simulink model "PMSM_FOC"  (R2015b)
settings: Solver=FixedStepDiscrete  StartTime=0.0  StopTime=0.3  RelTol=1e-3
PostLoadFcn:
  | PMSM_Params
undefined symbols (not defined in the file): Params, Plot_PMSM
libraries: powerlib x7
settings Model: Creator=Pascal  LastModifiedBy=reynaudp
settings DataIOCC: SaveFormat=Array
settings OptimizationCC: OptimizeModelRefInitCode=on  LifeSpan=1
settings DebuggingCC: UnderspecifiedInitializationDetection=Classic  MergeDetectMultiDrivingBlocksExec=none  SolverPrmCheckMsg=warning  StateNameClashWarn=warning
settings HardwareCC: ProdBitPerPointer=32  ProdLargestAtomicInteger=Integer  ProdWordSize=32  ProdHWDeviceType=STMicroelectronics->STM32 32-bit Cortex-M
settings RTWCC: SystemTargetFile=stm32.tlc  TemplateMakefile=stm32.tmf  Description=stm32 (Embedded Target)  GenerateReport=on  IncludeHyperlinkInReport=on  CodeExecutionProfiling=on  CodeProfilingSaveOptions=AllData  GenerateCodeReplacementReport=on
settings CodeAppCC: IgnoreCustomStorageClasses=off  MaxIdLength=64  CustomSymbolStrType=$N$R$M  SimulinkBlockComments=off  InternalIdentifier=Classic
settings STFCustomTargetCC: CodeReplacementLibrary=ARM CMSIS SIN COS  ParMdlRefBuildCompliant=on  ConcurrentExecutionCompliant=off  IncludeMdlTerminateFcn=off  GeneratePreprocessorConditionals=Use local settings  CombineOutputUpdateFcns=on  ERTCustomFileBanners=on  SupportContinuousTime=off  SupportNonInlinedSFcns=off  MATLABClassNameForMDSCustomization=Simulink.SoftwareTarget.ERTCustomization  CPPClassGenCompliant=off  GRTInterface=off  SystemTargetFile=stm32.tlc
settings ERTTargetCC: CodeReplacementLibrary=ARM CMSIS SIN COS  CompOptLevelCompliant=off  ConcurrentExecutionCompliant=off  IncludeMdlTerminateFcn=off  ERTFirstTimeCompliant=off  ModelStepFunctionPrototypeControlCompliant=off  CPPClassGenCompliant=off  UseToolchainInfoCompliant=off  ERTSrcFileBannerTemplate=sourceFileTemplate.cgt  ERTHdrFileBannerTemplate=sourceFileTemplate.cgt  ERTDataSrcFileTemplate=sourceFileTemplate.cgt  ERTDataHdrFileTemplate=sourceFileTemplate.cgt  ERTCustomFileTemplate=customRoutineProcess.tlc
settings ConfigComp: CovModelRefEnable=Off  CovSFcnEnable=off

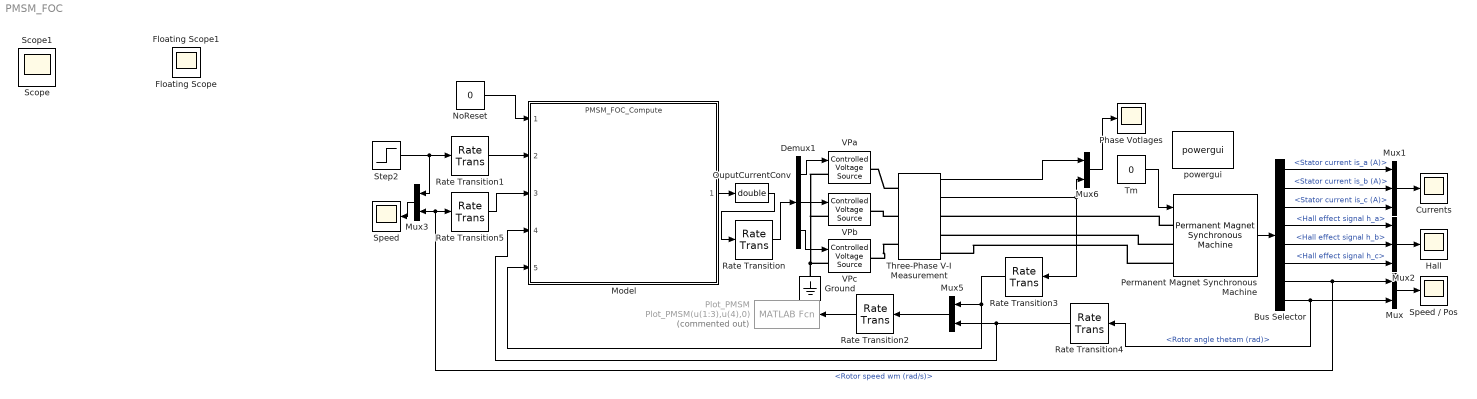
== system PMSM_FOC ==
  Bus Selector : BusSelector  OutputSignals=Stator current is_a (A),Stator current is_b (A),Stator current is_c (A),Hall effect signal h_a,Hall effect signal h_b,Hall effect signal h_c,Rotor speed wm (rad/s),Rotor angle thetam (rad)
  Currents : Scope
  Demux1 : Demux  Outputs=3
  Ground : powerlib/Elements/Ground  LConnTagsString=a
  Hall : Scope
  Model : ModelReference  ModelNameDialog=PMSM_FOC_Compute.slx  SimulationMode=Processor-in-the-loop (PIL)  ModelReferenceVersion=1.324  CopyOfModelName=PMSM_FOC_Compute.slx
  Mux{,3,5..6} (4 alike) : Mux  Inputs=2
  Mux1 : Mux  Inputs=3
  Mux2 : Mux  Inputs=3
  NoReset : Constant  Value=0  OutDataTypeStr=boolean
  OuputCurrentConv : DataTypeConversion  OutDataTypeStr=double
  Permanent Magnet Synchronous Machine : powerlib/Machines/Permanent Magnet Synchronous Machine  NbPhases=3  FluxDistribution=Sinusoidal  RotorType=Round  MechanicalLoad=Torque Tm  PresetModel=No  ShowDetailedParameters=on  MeasurementBus=off  Resistance=.6  Inductance=1.4e-3  dqInductances=[6e-4,6e-4]  La=1.4e-3  MachineConstant=Voltage Constant (V_peak L-L / krpm)  Flux=0.034182  VoltageCst=6.2  TorqueCst=0.051274  Flat=120  Mechanical=[1.1e-5,1e-4,1,0.02]  PolePairs=1  InitialConditions=[0,0 0,0]  InitialConditions5ph=[0 0 0 0 0 0]  TsPowergui=0  TsBlock=-1  RefAngle=Aligned with phase A axis (original Park)
  Phase Votlages : Scope
  Plot_PMSM : MATLABFcn  Commented=on  MATLABFcn=Plot_PMSM(u(1:3),u(4),0)  OutputDimensions=0  SampleTime=1/100
  Rate Transition{,1..5} (6 alike) : RateTransition
  Speed : Scope
  Speed / Pos : Scope
  Step2 : Step  Time=.01  After=130  SampleTime=0
  Three-Phase V-I Measurement : powerlib/Measurements/Three-Phase V-I Measurement  VoltageMeasurement=phase-to-ground  SetLabelV=off  LabelV=Vabc  Vpu=off  VpuLL=off  CurrentMeasurement=yes  SetLabelI=off  LabelI=Iabc  Ipu=off  Pbase=100e6  Vbase=500e3  OutputType=Complex  PhasorSimulation=off  PSBequivalent=0
  Tm : Constant  Value=0
  VPa : powerlib/Electrical Sources/Controlled Voltage Source  Initialize=on  Source_Type=AC  Amplitude=0  Phase=0  Frequency=0  Measurements=None
  VPb : powerlib/Electrical Sources/Controlled Voltage Source  Initialize=on  Source_Type=AC  Amplitude=0  Phase=0  Frequency=0  Measurements=None
  VPc : powerlib/Electrical Sources/Controlled Voltage Source  Initialize=on  Source_Type=AC  Amplitude=0  Phase=0  Frequency=0  Measurements=None
  powergui : powerlib/powergui  Priority=1  SimulationMode=Discrete  SolverType=Tustin  SampleTime=Params.T  frequency=60  SPID=off  DisableSnubberDevices=off  DisableRonSwitches=off  DisableVfSwitches=off  SwTol=0  DisplayEquations=off  Interpol=off  ExternalGateDelay=off  methode=off  Ts=0  FunctionMessages=off  echomessages=off  HookPort=off  EnableUseOfTLC=off  x0status=blocks  frequencyindice=0  Pbase=100e6  ErrMax=1e-4  Iterations=50  UnitsV=kV  UnitsW=MW  buscounter=0  RestoreLinks=warning  ResistiveCurrentMeasurement=off  Frange=[0:2:500]  Ylog=off  Xlog=on  ShowGrid=off  save=off  variable=ZData  structure=0  ZoomFFT=off  StartTime=0.0  cycles=1  DisplayStyle=1  fundamental=60  FreqAxis=off  MaxFrequency=1000  frequencyindicesteady=1  RmsSteady=1  display=off
  Floating Scope : Scope
  Floating Scope1 : Scope
  Scope : Scope
  Scope1 : Scope
  wires:
  Demux1/1 -> VPa/1
  Demux1/2 -> VPb/1
  Demux1/3 -> VPc/1
  Tm/1 -> Permanent Magnet Synchronous Machine/1
  Three-Phase V-I Measurement/1 -> Mux6/1
  Mux6/1 -> Phase Votlages/1
  Bus Selector/1 -> Mux1/1  "<Stator current is_a (A)>"
  Bus Selector/2 -> Mux1/2  "<Stator current is_b (A)>"
  Bus Selector/3 -> Mux1/3  "<Stator current is_c (A)>"
  Mux1/1 -> Currents/1
  Bus Selector/7 -> Mux/1, Mux3/2, Rate Transition5/1  "<Rotor speed wm (rad/s)>"
  Bus Selector/4 -> Mux2/1  "<Hall effect signal h_a>"
  Bus Selector/5 -> Mux2/2  "<Hall effect signal h_b>"
  Bus Selector/6 -> Mux2/3  "<Hall effect signal h_c>"
  Mux2/1 -> Hall/1
  Mux/1 -> Speed / Pos/1
  Permanent Magnet Synchronous Machine/1 -> Bus Selector/1
  Mux3/1 -> Speed/1
  Step2/1 -> Mux3/1, Rate Transition1/1
  Bus Selector/8 -> Mux/2, Rate Transition4/1  "<Rotor angle thetam (rad)>"
  Three-Phase V-I Measurement/2 -> Rate Transition3/1, Mux6/2
  Rate Transition1/1 -> Model/2
  Rate Transition5/1 -> Model/3
  Rate Transition4/1 -> Model/4, Mux5/2
  Mux5/1 -> Rate Transition2/1
  Rate Transition3/1 -> Model/5, Mux5/1
  Rate Transition2/1 -> Plot_PMSM/1
  NoReset/1 -> Model/1
  Model/1 -> OuputCurrentConv/1
  Rate Transition/1 -> Demux1/1
  OuputCurrentConv/1 -> Rate Transition/1
  connections:
  VPc/LConn1 -- VPb/LConn1 -- VPa/LConn1 -- Ground/LConn1
  Permanent Magnet Synchronous Machine/LConn1 -- Three-Phase V-I Measurement/RConn1
  Permanent Magnet Synchronous Machine/LConn2 -- Three-Phase V-I Measurement/RConn2
  Permanent Magnet Synchronous Machine/LConn3 -- Three-Phase V-I Measurement/RConn3
  Three-Phase V-I Measurement/LConn1 -- VPa/RConn1
  Three-Phase V-I Measurement/LConn2 -- VPb/RConn1
  Three-Phase V-I Measurement/LConn3 -- VPc/RConn1
